simulink model "GITvdp"  (R2014a)
settings: Solver=ode45  SolverMode=SingleTasking  StartTime=0.0  StopTime=20  RelTol=1e-3  AbsTol=1e-6
libraries: simulink x1
Description:
  | The van der Pol Equation
  | 
  | This is a simulation of a nonlinear second order system.
settings Model: ExtModeAutoUpdateStatusClock=off  Creator=The MathWorks Inc.  LastModifiedBy=sseshadr
settings DataIOCC: ExternalInput=[]  InitialState=[]  LimitDataPoints=off  SaveOutput=off  SaveTime=off
settings OptimizationCC: BlockReduction=off  BooleanDataType=off  InitFltsAndDblsToZero=on  BufferReusableBoundary=off
settings DebuggingCC: SaveWithParameterizedLinksMsg=none  UnderspecifiedInitializationDetection=Classic  SignalResolutionControl=TryResolveAllWithWarning  SolverPrmCheckMsg=none  MultiTaskDSMMsg=warning  MultiTaskCondExecSysMsg=none  FcnCallInpInsideContextMsg=UseLocalSettings  BusObjectLabelMismatch=none
settings HardwareCC: TargetUnknown=on
settings RTWCC: IncludeERTFirstTime=on
settings GRTTargetCC: TargetFcnLib=ansi_tfl_tmw.mat  CombineOutputUpdateFcns=off  GRTInterface=on

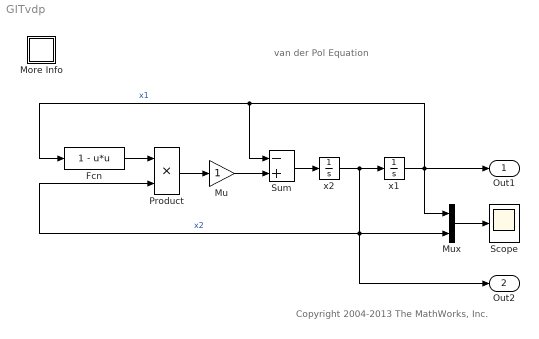
== system GITvdp ==
  note: van der Pol Equation
  note: Copyright 2004-2013 The MathWorks, Inc.
  Fcn : Fcn  Expr=1 - u*u
  More Info : Subsystem
      mask Display: disp('?')
  Mu : Gain  SaturateOnIntegerOverflow=on  OutDataTypeStr=Inherit: Same as input  ParamDataTypeStr=Inherit: Same as input
  Mux : Mux  Inputs=2
  Product : Product  SaturateOnIntegerOverflow=on  RndMeth=Zero  InputSameDT=on  OutDataTypeStr=Inherit: Same as first input
  Scope : Scope
      settings: TickLabels=on  TimeRange=20  YMin=-3  YMax=3
  Sum : Sum  Inputs=-+  SaturateOnIntegerOverflow=on  InputSameDT=on  OutDataTypeStr=Inherit: Same as first input
  x1 : Integrator  InitialCondition=2
  x2 : Integrator
  Out1 : Outport  InitialOutput=0
  Out2 : Outport  Port=2  InitialOutput=0
  wires:
  Sum/1 -> x2/1
  x2/1 -> Out2/1, Mux/2, Product/2, x1/1  "x2"
  x1/1 -> Out1/1, Mux/1, Fcn/1, Sum/1  "x1"
  Mux/1 -> Scope/1
  Product/1 -> Mu/1
  Mu/1 -> Sum/2
  Fcn/1 -> Product/1

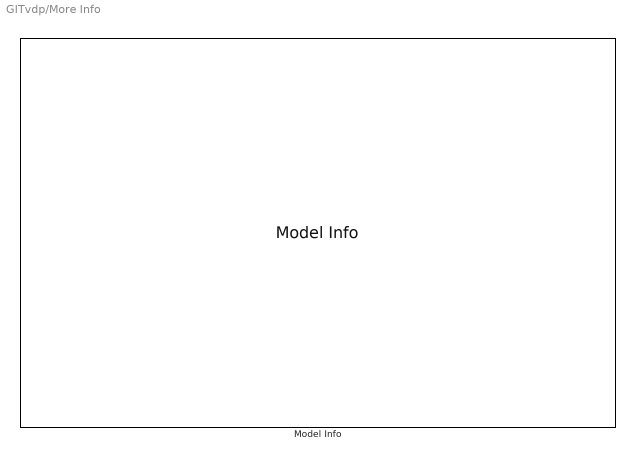
== system GITvdp/More Info ==
  Model Info : simulink/Model-Wide Utilities/Model Info  InitialBlockCM=None  BlockCM=None  Frame=on  DisplayStringWithTags=|  HorizontalTextAlignment=Left  LeftAlignmentValue=0.02  SourceBlockDiagram=vdp  TagMaxNumber=20
      | Model Description:
      | -------------------
      | 
      | %<Description>
